simulink model "LoadFlow116BusNetwork_original"  (R2024a)
settings: Solver=FixedStepDiscrete  StartTime=0.0  StopTime=4.5  FixedStep=75e-6  RelTol=1e-3  EnableMultiTasking=on
undefined symbols (not defined in the file or in its folder): D1, D11, Delta
libraries: spsSeriesRLCBranchLib x164, spsLoadFlowBusLib x116, spsDistributedParametersLineLib x79, spsThreePhaseSeriesRLCLoadLib x60, spsThreePhaseTransformerTwoWindingsLib x52, spsThreePhaseParallelRLCLoadLib x44, spsThreePhaseVIMeasurementLib x44, spsSynchronousMachinepuStandardLib x28, spsExcitationSystemLib x28, spsHydraulicTurbineandGovernorLib x28, spsGenericPowerSystemStabilizerLib x28, spsMultiBandPowerSystemStabilizerLib x28
(part 8 of 15)

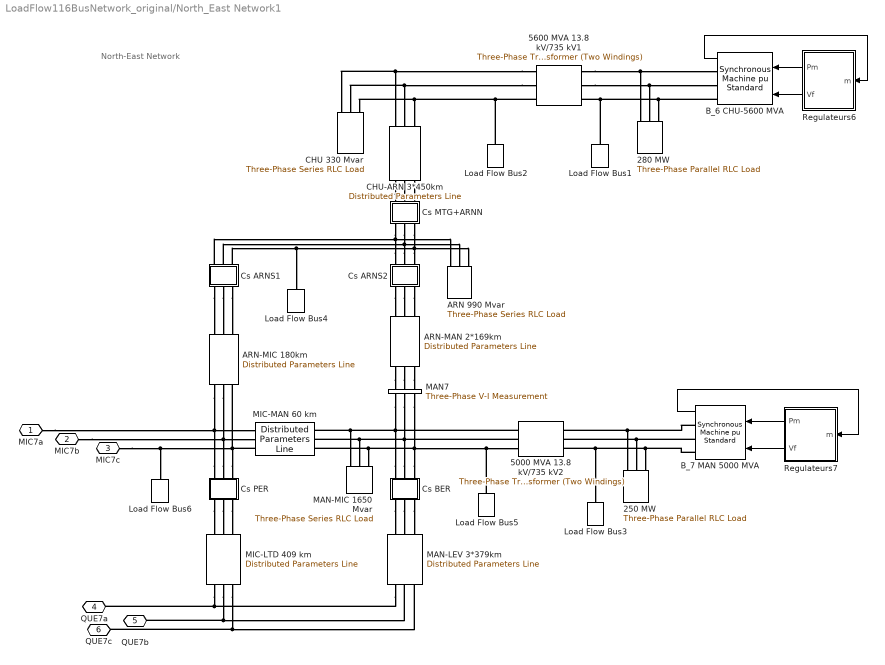
== system LoadFlow116BusNetwork_original/North_East Network1 ==
  note: North-East Network
  250 MW : spsThreePhaseParallelRLCLoadLib/Three-Phase Parallel RLC Load  LConnTagsString=A|B|C  Configuration=Y (grounded)  NominalVoltage=(13800)*1  Vabc=[1e3 1e3 1e3]  Vabcp=[1e3 1e3 1e3]  NominalFrequency=60  UnbalancedPower=off  ActivePower=250000000  InductivePower=0  CapacitivePower=0  Pabc=[10e3 9e3 11e3]  QLabc=[100 90 110]  QCabc=[100 90 110]  Pabcp=[10e3 9e3 11e3]  QLabcp=[100 90 110]  QCabcp=[100 90 110]  Measurements=None  LoadType=constant PQ
  280 MW : spsThreePhaseParallelRLCLoadLib/Three-Phase Parallel RLC Load  LConnTagsString=A|B|C  Configuration=Y (grounded)  NominalVoltage=(13800)*1  Vabc=[1e3 1e3 1e3]  Vabcp=[1e3 1e3 1e3]  NominalFrequency=60  UnbalancedPower=off  ActivePower=280000000  InductivePower=0  CapacitivePower=0  Pabc=[10e3 9e3 11e3]  QLabc=[100 90 110]  QCabc=[100 90 110]  Pabcp=[10e3 9e3 11e3]  QLabcp=[100 90 110]  QCabcp=[100 90 110]  Measurements=None  LoadType=constant PQ
  5000 MVA 13.8 kV/735 kV2 : spsThreePhaseTransformerTwoWindingsLib/Three-Phase Transformer (Two Windings)  Winding1Connection=Delta (D1)  Winding2Connection=Yg  CoreType=Three single-phase transformers  SetSaturation=off  Hysteresis=off  DataFile='basic_model'  SetInitialFlux=off  Measurements=None  UNITS=pu  NominalPower=[ 5000e6 60 ]  Winding1="[ 13.8e3 0.002  0.0]"  Winding2=[ 735e3 0.002 0.12]  Rm=500  Lm=500  L0=0.5  Saturation="[ 0,0  ;  0.005,1.2  ;  1.0,1.4 ]"  InitialFluxes=[ 0.8 , -0.8 , 0.7 ]  BreakLoop=off  DiscreteSolver=Trapezoidal iterative  DataType=off  TransfoNumber=0
  5600 MVA 13.8 kV/735 kV1 : spsThreePhaseTransformerTwoWindingsLib/Three-Phase Transformer (Two Windings)  Winding1Connection=Delta (D1)  Winding2Connection=Yg  CoreType=Three single-phase transformers  SetSaturation=off  Hysteresis=off  DataFile='basic_model'  SetInitialFlux=off  Measurements=None  UNITS=pu  NominalPower=[ 5600e6 60 ]  Winding1="[ 13.8e3 0.002  0.0]"  Winding2=[ 735e3 0.002 0.12]  Rm=500  Lm=500  L0=0.5  Saturation="[ 0,0  ;  0.005,1.2  ;  1.0,1.4 ]"  InitialFluxes=[ 0.8 , -0.8 , 0.7 ]  BreakLoop=off  DiscreteSolver=Trapezoidal iterative  DataType=off  TransfoNumber=0
  ARN 990 Mvar : spsThreePhaseSeriesRLCLoadLib/Three-Phase Series RLC Load  LConnTagsString=A|B|C  Configuration=Y (grounded)  NominalVoltage=735e3  Vabc=[1e3 1e3 1e3]  Vabcp=[1e3 1e3 1e3]  NominalFrequency=60  UnbalancedPower=off  ActivePower=3300000  InductivePower=990e6  CapacitivePower=0  Pabc=[10e3 9e3 11e3]  QLabc=[100 90 110]  QCabc=[100 90 110]  Pabcp=[10e3 9e3 11e3]  QLabcp=[100 90 110]  QCabcp=[100 90 110]  Measurements=None  LoadType=constant Z
  ARN-MAN 2*169km : spsDistributedParametersLineLib/Distributed Parameters Line  Phases=3  Length=169  Frequency=60  Resistance="[0.01273  0.3864]/2"  Inductance="[0.9337e-3  4.1264e-3]/2"  Capacitance=[12.74e-9 7.751e-9]*2  x1=[-0.000975 8.78499508384115e-10 336881.671287458 -573361.279314323;-0.0009 8.13651182104684e-10 352956.287913021 -563608.347624883;-0.000825 7.4815243551956e-10 368748.756682439 -553404.876045849;-0.00075 6.82055627324597e-10 384246.453337811 -542759.021076282;-0.000675 6.15413594296952e-10 399436.989257552 -531679.292849758;-0.0006 5.48279609058169e-10 414308.221359671 -520174.548331497;-0.000525 4.80707337488865e-10 428848.261808764 -508253.984238236;-0.00045 4.12750795829041e-10 443045.487518965 -495927.129686522;-0.000375 3.44464307498331e-10 456888.549445267 -483203.838575277;-0.0003 2.75902459670687e-10 470366.381655772 -470094.281708741;-0.000225 2.07120059638231e-10 483468.210177628 -456608.93866609;-0.00015 1.38172090999144e-10 496183.56160958 -442758.589424221;-7.5e-05 6.91136697046154e-11 508502.271494244 -428554.3057404]  x2=[-0.000975 3.53873333334227e-10 221203.742399991 -593985.664844307;-0.0009 3.00275393624317e-10 237907.645286788 -587494.731105826;-0.000825 2.46437418359111e-10 254421.368442051 -580534.163068269;-0.00075 1.92402444792288e-10 270731.71104816 -573109.524903227;-0.000675 1.38213667654954e-10 286825.63486679 -565226.751752846;-0.0006 8.39144046264366e-11 302690.274661488 -556892.144985374;-0.000525 2.95480617067942e-11 318312.948481937 -548112.367157935;-0.00045 -2.4841901481276e-11 333681.167801722 -538894.436690592;-0.000375 -7.9212006433396e-11 348782.647501459 -529245.722255919;-0.0003 -1.33518790519557e-10 363605.315689336 -519173.936888605;-0.000225 -1.87718841727484e-10 378137.3233512 -508687.131819771;-0.00015 -2.41768833365527e-10 392367.053822471 -497793.690040934;-7.5e-05 -2.95625558697366e-10 406283.132074335 -486502.319602777]  x3=[-0.000975 -3.60869348928103e-12 1173.57899596787 -608.93138738685;-0.0009 -3.82766651260744e-12 1190.32360835435 -575.511145378701;-0.000825 -4.04357975788894e-12 1206.11669426088 -541.630848566551;-0.00075 -4.25626062738083e-12 1220.94562893621 -507.317580341287;-0.000675 -4.46553910725016e-12 1234.79855835687 -472.598770204517;-0.0006 -4.6712479034822e-12 1247.66440870303 -437.50217184185;-0.000525 -4.87322257561268e-12 1259.53289521077 -402.05584093702;-0.00045 -5.07130166817902e-12 1270.39453039359 -366.288112744606;-0.000375 -5.26532683978534e-12 1280.2406316265 -330.227579439259;-0.0003 -5.45514298967813e-12 1289.06332808682 -293.903067259561;-0.000225 -5.64059838173146e-12 1296.855567046 -257.343613464762;-0.00015 -5.82154476574249e-12 1303.61111950744 -220.57844312285;-7.5e-05 -5.9978374959404e-12 1309.32458518586 -183.636945748468]  x4=[-0.000975 4.09065354206605e-12 1977.23728446549 -8416.68856749933;-0.0009 4.02816421017437e-12 2214.39295528562 -8357.4267304651;-0.000825 3.96245482544606e-12 2449.77847425865 -8291.48409437546;-0.00075 3.89357791495788e-12 2683.20567780222 -8218.91337276473;-0.000675 3.82158853785822e-12 2914.48796778139 -8139.77257755741;-0.0006 3.74654424135366e-12 3143.44046067226 -8054.12497269428;-0.000525 3.66850501470661e-12 3369.88013535513 -7962.03902356022;-0.00045 3.58753324128082e-12 3593.62597941869 -7863.58834225402;-0.000375 3.50369364867304e-12 3814.49913385863 -7758.85162874395;-0.0003 3.41705325697083e-12 4032.32303605475 -7647.91260795627;-0.000225 3.32768132517766e-12 4246.92356091246 -7530.85996284678;-0.00015 3.23564929584838e-12 4458.12916005569 -7407.78726350902;-7.5e-05 3.14103073797909e-12 4665.77099896003 -7278.79289237575]  x5=0.000955765248222805  V1=ones(3,3)  V2=ones(3,3)  I1=ones(3,3)  I2=ones(3,3)  nHarmo=1  Measurements=None  Decoupling=off  VsMag0=[ 1 1 1]  VrMag0=[ 1 1 1]  VsAngle0=[0 -120 120]  VrAngle0=[0 -120 120]  IsMag0=[ 1 1 1]  IrMag0=[ 1 1 1]  IsAngle0=[0 -120 120]  IrAngle0=[0 -120 120]
      settings: AttributesFormatString=\n  LibrarySourceBlock=sps_lib/Power Grid Elements/Distributed Parameters Line
  ARN-MIC 180km : spsDistributedParametersLineLib/Distributed Parameters Line  Phases=3  Length=180  Frequency=60  Resistance="[0.01273  0.3864]"  Inductance="[0.9337e-3  4.1264e-3]"  Capacitance=[12.74e-9 7.751e-9]  x1=[-0.00105 5.00976431216861e-10 327893.271560114 -568370.375306689;-0.000975 4.5408234490734e-10 343830.386178249 -558873.543002063;-0.0009 4.06825272118994e-10 359492.648046455 -548929.955738212;-0.000825 3.5924298943275e-10 374867.536992234 -538547.562266654;-0.00075 3.11373533397356e-10 389942.762564607 -527734.662113874;-0.000675 2.63255170123539e-10 404706.273858911 -516499.898946812;-0.0006 2.14926364694664e-10 419146.269150106 -504852.253663245;-0.000525 1.66425750418337e-10 433251.205326894 -492801.037212598;-0.00045 1.17792097943524e-10 447009.807119111 -480355.883152912;-0.000375 6.90642842678944e-11 460411.076110995 -467526.739949925;-0.0003 2.02812616601402e-11 473444.299533163 -454323.863024421;-0.000225 -2.85179734778713e-11 486099.058826224 -440757.806554203;-0.00015 -7.72944117842243e-11 498365.237969224 -426839.415037247;-7.5e-05 -1.26009062120441e-10 510233.031566236 -412579.814622772]  x2=[-0.00105 2.18032175619013e-09 183777.347501384 -621430.397175494;-0.000975 2.1855909220691e-09 201272.089254416 -615986.559734681;-0.0009 2.18911296000564e-09 218605.937178865 -610050.312062926;-0.000825 2.19088505453651e-09 235765.034861915 -603626.399505791;-0.00075 2.19090578907644e-09 252735.665583423 -596719.957240685;-0.000675 2.18917514705056e-09 269504.263280849 -589336.506171882;-0.0006 2.18569451190764e-09 286057.423393762 -581481.948517196;-0.000525 2.18046666601414e-09 302381.913579239 -573162.563089837;-0.00045 2.1734957884301e-09 318464.6842896 -564385.000279226;-0.000375 2.16478745156838e-09 334292.879204012 -555156.276734772;-0.0003 2.15434861674024e-09 349853.845505641 -545483.769756872;-0.000225 2.14218762859051e-09 365135.143996117 -535375.21139961;-0.00015 2.12831420842706e-09 380124.559039236 -524838.68228987;-7.5e-05 2.11273944644969e-09 394810.108325961 -513882.605167809]  x3=[-0.00105 -4.40575400200817e-12 35.6370942882288 24.8424671154528;-0.000975 -4.25272459462188e-12 34.9200556849036 25.839604901741;-0.0009 -4.09629562426352e-12 34.1751025233587 26.81608690323;-0.000825 -3.93659213785855e-12 33.4028303077532 27.7711325351485;-0.00075 -3.77374179993046e-12 32.6038563806801 28.7039783486309;-0.000675 -3.60787479054769e-12 31.778819429672 29.613878641007;-0.0006 -3.43912370125969e-12 30.9283789766441 30.500106051905;-0.000525 -3.26762342910525e-12 30.0532148506823 31.3619521446925;-0.00045 -3.09351106877791e-12 29.1540266445985 32.1987279727894;-0.000375 -2.91692580303449e-12 28.2315331556866 33.0097646304019;-0.0003 -2.73800879143459e-12 27.286471811127 33.7944137872352;-0.000225 -2.55690305749976e-12 26.3195980784985 34.5520482067589;-0.00015 -2.37375337438269e-12 25.3316848618695 35.2820622476101;-7.5e-05 -2.18870614913778e-12 24.3235218839497 35.9838723477343]  x4=[-0.00105 7.31127026918303e-12 1327.91429807013 -4613.1254825023;-0.000975 7.11574515856379e-12 1457.79983330337 -4573.74071492959;-0.0009 6.91453183013935e-12 1586.52002565494 -4530.69976900994;-0.000825 6.70779113076577e-12 1713.97197817258 -4484.03705101698;-0.00075 6.49568832579491e-12 1840.05380771551 -4433.7898624135;-0.000675 6.27839296696377e-12 1964.66472639833 -4379.99837003327;-0.0006 6.05607875685747e-12 2087.70512215924 -4322.70557397225;-0.000525 5.82892341005406e-12 2209.07663838846 -4261.95727321502;-0.00045 5.59710851106216e-12 2328.68225255295 -4197.80202902371;-0.000375 5.36081936916516e-12 2446.42635375479 -4130.29112611892;-0.0003 5.12024487028773e-12 2562.21481916101 -4059.47853168349;-0.000225 4.87557732600336e-12 2675.955089244 -3985.42085222194;-0.00015 4.62701231980343e-12 2787.55624177213 -3908.1772883101;-7.5e-05 4.3747485507507e-12 2896.92906449163 -3827.8095872711]  x5=0.00101797482059234  V1=ones(3,3)  V2=ones(3,3)  I1=ones(3,3)  I2=ones(3,3)  nHarmo=1  Measurements=None  Decoupling=off  VsMag0=[ 1 1 1]  VrMag0=[ 1 1 1]  VsAngle0=[0 -120 120]  VrAngle0=[0 -120 120]  IsMag0=[ 1 1 1]  IrMag0=[ 1 1 1]  IsAngle0=[0 -120 120]  IrAngle0=[0 -120 120]
      settings: AttributesFormatString=\n  LibrarySourceBlock=sps_lib/Power Grid Elements/Distributed Parameters Line
  "B_6 CHU-5600 MVA " : spsSynchronousMachinepuStandardLib/Synchronous Machine pu Standard  PresetModel=No  MechanicalLoad=Mechanical power Pm  ShowDetailedParameters=on  RotorType=Salient-pole  Units=per unit standard parameters  MeasurementBus=off  NominalParameters="[ 5600E6  13800   60 ]"  Reactances1=[ 31 32 33 34 35 36 37 ]  Reactances2=[ 1.305, 0.296, 0.252, 0.474, 0.243, 0.18 ]  dAxisTimeConstants=Short-circuit  qAxisTimeConstants=Open-circuit  TimeConstants1=[]  TimeConstants2=[]  TimeConstants3=[]  TimeConstants4=[]  TimeConstants5=[ 1.01, 0.053, 0.1 ]  TimeConstants6=[]  TimeConstants7=[]  TimeConstants8=[]  StatorResistance=2.8544e-3  Mechanical="[ 4.0 0  32]"  PolePairs=32  InitialConditions=[0 -61.7964 0.894782 0.894782 0.894782 8.48442 -111.516 128.484 1.31361]  SetSaturation=off  Saturation=[0.6404,0.7127,0.8441,0.9214,0.9956,1.082,1.19,1.316,1.457;0.7,0.7698,0.8872,0.9466,0.9969,1.046,1.1,1.151,1.201]  LoadFlowParameters=[1 5000000000 0 0 0]  TsPowergui=0  TsBlock=-1  IterativeModel=Trapezoidal non iterative  IterativeDiscreteModel=Trapezoidal non iterative  BusType=PV  Pref=5000000000  Qref=0  Qmin=-Inf  Qmax=Inf  PLF=0  QLF=0
  B_7 MAN 5000 MVA : spsSynchronousMachinepuStandardLib/Synchronous Machine pu Standard  PresetModel=No  MechanicalLoad=Mechanical power Pm  ShowDetailedParameters=on  RotorType=Salient-pole  Units=per unit standard parameters  MeasurementBus=off  NominalParameters="[ 5000E6  13800   60 ]"  Reactances1=[ 31 32 33 34 35 36 37 ]  Reactances2=[ 1.305, 0.296, 0.252, 0.474, 0.243, 0.18 ]  dAxisTimeConstants=Short-circuit  qAxisTimeConstants=Open-circuit  TimeConstants1=[]  TimeConstants2=[]  TimeConstants3=[]  TimeConstants4=[]  TimeConstants5=[ 1.01, 0.053, 0.1 ]  TimeConstants6=[]  TimeConstants7=[]  TimeConstants8=[]  StatorResistance=2.8544e-3  Mechanical="[ 3.7 0  32]"  PolePairs=32  InitialConditions=[0 -81.9543 0.907703 0.907703 0.907703 -8.76021 -128.76 111.24 1.25655]  SetSaturation=off  Saturation=[0.6404,0.7127,0.8441,0.9214,0.9956,1.082,1.19,1.316,1.457;0.7,0.7698,0.8872,0.9466,0.9969,1.046,1.1,1.151,1.201]  LoadFlowParameters=[1 4500000000 0 0 0]  TsPowergui=0  TsBlock=-1  IterativeModel=Trapezoidal non iterative  IterativeDiscreteModel=Trapezoidal non iterative  BusType=PV  Pref=4500000000  Qref=0  Qmin=-Inf  Qmax=Inf  PLF=0  QLF=0
  CHU 330 Mvar : spsThreePhaseSeriesRLCLoadLib/Three-Phase Series RLC Load  LConnTagsString=A|B|C  Configuration=Y (grounded)  NominalVoltage=735e3  Vabc=[1e3 1e3 1e3]  Vabcp=[1e3 1e3 1e3]  NominalFrequency=60  UnbalancedPower=off  ActivePower=1100000  InductivePower=330e6  CapacitivePower=0  Pabc=[10e3 9e3 11e3]  QLabc=[100 90 110]  QCabc=[100 90 110]  Pabcp=[10e3 9e3 11e3]  QLabcp=[100 90 110]  QCabcp=[100 90 110]  Measurements=None  LoadType=constant Z
  CHU-ARN 3*450km : spsDistributedParametersLineLib/Distributed Parameters Line  Phases=3  Length=450  Frequency=60  Resistance="[0.01273  0.3864]/3"  Inductance="[0.9337e-3  4.1264e-3]/3"  Capacitance=[12.74e-9 7.751e-9]*3  x1=[-0.00255 7.32999303821091e-10 0 0;-0.002475 6.56025529209857e-10 0 0;-0.0024 5.785273378281e-10 0 0;-0.002325 5.00566680544248e-10 0 0;-0.00225 4.22205877914896e-10 0 0;-0.002175 3.43507570366705e-10 0 0;-0.0021 2.64534668122606e-10 0 0;-0.002025 1.85350300912325e-10 0 0;-0.00195 1.0601776750745e-10 0 0;-0.001875 2.66004851213558e-11 0 0;-0.0018 -5.28380612855433e-11 0 0;-0.001725 -1.32234369754701e-10 0 0;-0.00165 -2.1152497209193e-10 0 0;-0.001575 -2.90646484602909e-10 351966.370721056 -543333.024589183;-0.0015 -3.69535658761137e-10 367186.081536598 -533165.672906027;-0.001425 -4.48129431767837e-10 382112.269416695 -522572.116741658;-0.00135 -5.26364976963391e-10 396733.002595135 -511560.824422788;-0.001275 -6.04179754050015e-10 411036.593481518 -500140.598208017;-0.0012 -6.81511559085512e-10 425011.608004143 -488320.567251446;-0.001125 -7.58298574208153e-10 438646.874750225 -476110.18030497;-0.00105 -8.34479417052929e-10 451931.493896154 -463519.198165088;-0.000975 -9.09993189819675e-10 464854.845920646 -450557.685870274;-0.0009 -9.84779527953843e-10 477406.600093827 -437236.00465514;-0.000825 -1.058778648401e-09 489576.722735458 -423564.803667819;-0.00075 -1.13193139739647e-09 501355.48523571 -409555.011457205;-0.000675 -1.20417929775201e-09 512733.471832061 -395217.827236834;-0.0006 -1.27546459560147e-09 523701.587136114 -380564.711932406;-0.000525 -1.34573030656848e-09 534251.063404314 -365607.379020094;-0.00045 -1.41492026131878e-09 544373.467546744 -350357.785162973;-0.000375 -1.48297915046119e-09 554060.70786841 -334828.120653048;-0.0003 -1.54985256876106e-09 563305.04053762 -319030.799666514;-0.000225 -1.61548705863101e-09 572099.075776279 -302978.450340062;-0.00015 -1.67983015286406e-09 580435.783767173 -286683.904676134;-7.5e-05 -1.74283041657518e-09 588308.500273488 -270160.188285219]  x2=[-0.00255 1.95007004339389e-09 0 0;-0.002475 1.90177200864104e-09 0 0;-0.0024 1.85195372644257e-09 0 0;-0.002325 1.80065502077103e-09 0 0;-0.00225 1.74791689902682e-09 0 0;-0.002175 1.69378151925756e-09 0 0;-0.0021 1.63829215645754e-09 0 0;-0.002025 1.58149316797435e-09 0 0;-0.00195 1.52342995805033e-09 0 0;-0.001875 1.46414894152712e-09 0 0;-0.0018 1.40369750674227e-09 0 0;-0.001725 1.34212397764783e-09 0 0;-0.00165 1.27947757518084e-09 0 0;-0.001575 1.21580837791692e-09 34511.8097316182 -640486.415414582;-0.0015 1.15116728203818e-09 52604.9373492512 -639254.768695381;-0.001425 1.08560596064763e-09 70656.0133848497 -637512.111495011;-0.00135 1.01917682246247e-09 88650.6080844217 -635259.836866974;-0.001275 9.51932969919355e-10 106574.336844291 -632499.745245147;-0.0012 8.83928156725153e-10 124412.871709928 -629234.043004542;-0.001125 8.15216744887019e-10 142151.952829502 -625465.340697562;-0.00105 7.45853661256256e-10 159777.399852982 -621196.65096717;-0.000975 6.75894353620629e-10 177275.123267695 -616431.386138622;-0.0009 6.05394746380248e-10 194631.135661268 -611173.355491711;-0.000825 5.34411195842461e-10 211831.56290295 -605426.762215686;-0.00075 4.63000445171483e-10 228862.655234379 -599196.200049286;-0.000675 3.91219579028779e-10 245710.79826093 -592486.649608576;-0.0006 3.1912597794046e-10 262362.523834852 -585303.474405518;-0.000525 2.46777272428167e-10 278804.520821502 -577652.416560464;-0.00045 1.74231296940113e-10 295023.645740059 -569539.592211991;-0.000375 1.01546043619113e-10 311006.933270225 -560971.48662775;-0.0003 2.87796159445515e-11 326741.6066165 -551954.949020251;-0.000225 -4.40098177146536e-11 342215.087721761 -542497.1870717;-0.00015 -1.1676407059895e-10 357415.007321963 -532605.761172288;-7.5e-05 -1.89424984071761e-10 372329.214833944 -522288.578376537]  x3=[-0.00255 4.87239052788349e-12 0 0;-0.002475 4.7899343714918e-12 0 0;-0.0024 4.703649214852e-12 0 0;-0.002325 4.61360403299809e-12 0 0;-0.00225 4.51987080667071e-12 0 0;-0.002175 4.42252446477682e-12 0 0;-0.0021 4.32164282449269e-12 0 0;-0.002025 4.217306529058e-12 0 0;-0.00195 4.10959898331094e-12 0 0;-0.001875 3.99860628701559e-12 0 0;-0.0018 3.88441716603514e-12 0 0;-0.001725 3.76712290140572e-12 0 0;-0.00165 3.64681725636784e-12 0 0;-0.001575 3.52359640141339e-12 -94.8473576352802 -855.378108345468;-0.0015 3.39755883740849e-12 -70.6281637624271 -857.719458194341;-0.001425 3.26880531685335e-12 -46.3525108161095 -859.375160231881;-0.00135 3.13743876334233e-12 -22.0398043818627 -860.343890915213;-0.001275 3.0035641892883e-12 2.29052033478661 -860.62487585585;-0.0012 2.86728861197744e-12 26.6190140445265 -860.21789043873;-0.001125 2.72872096802114e-12 50.9262289217237 -859.123260001768;-0.00105 2.58797202627384e-12 75.1927341507184 -857.341859575788;-0.000975 2.44515429928604e-12 99.3991314585203 -854.875113185033;-0.0009 2.3003819533635e-12 123.526070621492 -851.724992708825;-0.000825 2.15377071730447e-12 147.554264933621 -847.894016305276;-0.00075 2.00543778988782e-12 171.464506624018 -843.385246398306;-0.000675 1.85550174618617e-12 195.237682211315 -838.202287229592;-0.0006 1.70408244277874e-12 218.854787782689 -832.349281977391;-0.000525 1.55130092193989e-12 242.2969441853 -825.830909444549;-0.00045 1.39727931487974e-12 265.545412117997 -818.652380318334;-0.000375 1.24214074411436e-12 288.581607111227 -810.819433005094;-0.0003 1.08600922504354e-12 311.38711438318 -802.338329043062;-0.000225 9.29009566814706e-13 333.943703560277 -793.215848096982;-0.00015 7.71267272552487e-13 356.233343250259 -783.459282538543;-7.5e-05 6.12908439033376e-13 378.238215456199 -773.076431616971]  x4=[-0.00255 1.21136319031042e-11 0 0;-0.002475 1.18418780553791e-11 0 0;-0.0024 1.15606579915234e-11 0 0;-0.002325 1.12701965145533e-11 0 0;-0.00225 1.09707258149292e-11 0 0;-0.002175 1.06624852849464e-11 0 0;-0.0021 1.03457213273683e-11 0 0;-0.002025 1.00206871584559e-11 0 0;-0.00195 9.68764260555077e-12 0 0;-0.001875 9.34685389937263e-12 0 0;-0.0018 8.99859346119899e-12 0 0;-0.001725 8.64313968509556e-12 0 0;-0.00165 8.28077671537234e-12 0 0;-0.001575 7.91179421944299e-12 398.583364809259 -13326.9833161388;-0.0015 7.53648715626912e-12 775.187270557429 -13310.3877177131;-0.001425 7.15515554057465e-12 1151.17150346228 -13283.1519990016;-0.00135 6.76810420301859e-12 1526.23550748077 -13245.2979318211;-0.001275 6.37564254651811e-12 1900.07946218677 -13196.8557761338;-0.0012 5.97808429891655e-12 2272.40452244289 -13137.8642558577;-0.001125 5.57574726219419e-12 2642.91305729273 -13068.3705279116;-0.00105 5.16895305842222e-12 3011.30888788249 -12988.4301445182;-0.000975 4.75802687266299e-12 3377.29752422184 -12898.1070087969;-0.0009 4.343297193022e-12 3740.58640059472 -12797.4733236804;-0.000825 3.92509554805959e-12 4100.88510943186 -12686.6095341969;-0.00075 3.50375624177203e-12 4457.90563345816 -12565.6042631634;-0.000675 3.07961608635407e-12 4811.36257592932 -12434.5542403421;-0.0006 2.65301413295638e-12 5160.9733887736 -12293.5642251162;-0.000525 2.22429140065329e-12 5506.45859845643 -12142.7469227465;-0.00045 1.79379060383731e-12 5847.5420293873 -11982.222894277;-0.000375 1.36185587825854e-12 6183.95102469027 -11812.12046016;-0.0003 9.28832505927784e-13 6515.41666416172 -11632.5755976787;-0.000225 4.95066639103405e-13 6841.67397924106 -11443.731832249;-0.00015 6.09050235824992e-14 7162.46216482252 -11245.7401226875;-7.5e-05 -3.7330527848238e-13 7477.52478773877 -11038.7587405375]  x5=0.00254493705148084  V1=ones(3,3)  V2=ones(3,3)  I1=ones(3,3)  I2=ones(3,3)  nHarmo=1  Measurements=None  Decoupling=off  VsMag0=[ 1 1 1]  VrMag0=[ 1 1 1]  VsAngle0=[0 -120 120]  VrAngle0=[0 -120 120]  IsMag0=[ 1 1 1]  IrMag0=[ 1 1 1]  IsAngle0=[0 -120 120]  IrAngle0=[0 -120 120]
      settings: AttributesFormatString=\n  LibrarySourceBlock=sps_lib/Power Grid Elements/Distributed Parameters Line
  "Cs ARNS1 " : Subsystem  mask{Xc=25}
      mask prompts: Xc "Condensator Reactance at  60Hz  (ohm):"
      mask help: Series Compensation
      mask init:
      | Cs=1/Xc/(2*pi*60);
      mask Display: disp('Cs')
  Cs ARNS2 : Subsystem  mask{Xc=25/2}
      mask prompts: Xc "Condensator Reactance at  60Hz  (ohm):"
      mask help: Series Compensation
      mask init:
      | Cs=1/Xc/(2*pi*60);
      mask Display: disp('Cs')
  Cs BER : Subsystem  mask{Xc=22/3}
      mask prompts: Xc "Condensator Reactance at  60Hz  (ohm):"
      mask help: Series Compensation
      mask init:
      | Cs=1/Xc/(2*pi*60);
      mask Display: disp('Cs')
  "Cs MTG+ARNN " : Subsystem  mask{Xc=(30+25)/3}
      mask prompts: Xc "Condensator Reactance at  60Hz  (ohm):"
      mask help: Series Compensation
      mask init:
      | Cs=1/Xc/(2*pi*60);
      mask Display: disp('Cs')
  "Cs PER " : Subsystem  mask{Xc=22}
      mask prompts: Xc "Condensator Reactance at  60Hz  (ohm):"
      mask help: Series Compensation
      mask init:
      | Cs=1/Xc/(2*pi*60);
      mask Display: disp('Cs')
  Load Flow Bus1 : spsLoadFlowBusLib/Load Flow Bus  LConnTagsString=a  Phases=single  Connectors=on one side  ID=CHU_13.8  Vbase=13.8e3  Vref=1  Vangle=0  VLF=1  VLFb=1  VLFc=1  angleLF=4.726  angleLFb=0  angleLFc=0
      settings: AttributesFormatString=%<ID>\n%<Vbase>V\n%<VLF>pu\n%<angleLF>deg.
  Load Flow Bus2 : spsLoadFlowBusLib/Load Flow Bus  LConnTagsString=a  Phases=single  Connectors=on one side  ID=CHU7  Vbase=735e3  Vref=1  Vangle=0  VLF=1.009  VLFb=1  VLFc=1  angleLF=28.97  angleLFb=0  angleLFc=0
      settings: AttributesFormatString=%<ID>\n%<Vbase>V\n%<VLF>pu\n%<angleLF>deg.
  Load Flow Bus3 : spsLoadFlowBusLib/Load Flow Bus  LConnTagsString=a  Phases=single  Connectors=on one side  ID=MAN_13.8  Vbase=13.8e3  Vref=1  Vangle=0  VLF=1  VLFb=1  VLFc=1  angleLF=-16.23  angleLFb=0  angleLFc=0
      settings: AttributesFormatString=%<ID>\n%<Vbase>V\n%<VLF>pu\n%<angleLF>deg.
  Load Flow Bus4 : spsLoadFlowBusLib/Load Flow Bus  LConnTagsString=a  Phases=single  Connectors=on one side  ID=ARN7  Vbase=735e3  Vref=1  Vangle=0  VLF=1.054  VLFb=1  VLFc=1  angleLF=12.72  angleLFb=0  angleLFc=0
      settings: AttributesFormatString=%<ID>\n%<Vbase>V\n%<VLF>pu\n%<angleLF>deg.
  Load Flow Bus5 : spsLoadFlowBusLib/Load Flow Bus  LConnTagsString=a  Phases=single  Connectors=on one side  ID=MAN7  Vbase=735e3  Vref=1  Vangle=0  VLF=1.016  VLFb=1  VLFc=1  angleLF=7.996  angleLFb=0  angleLFc=0
      settings: AttributesFormatString=%<ID>\n%<Vbase>V\n%<VLF>pu\n%<angleLF>deg.
  Load Flow Bus6 : spsLoadFlowBusLib/Load Flow Bus  LConnTagsString=a  Phases=single  Connectors=on one side  ID=MIC7  Vbase=735e3  Vref=1  Vangle=0  VLF=1.041  VLFb=1  VLFc=1  angleLF=5.981  angleLFb=0  angleLFc=0
      settings: AttributesFormatString=%<ID>\n%<Vbase>V\n%<VLF>pu\n%<angleLF>deg.
  MAN-LEV 3*379km : spsDistributedParametersLineLib/Distributed Parameters Line  Phases=3  Length=379  Frequency=60  Resistance="[0.01273  0.3864]/3"  Inductance="[0.9337e-3  4.1264e-3]/3"  Capacitance=[12.74e-9 7.751e-9]*3  x1=[-0.002175 1.67803313912777e-09 2062.1369044793 -628964.364618995;-0.0021 1.66910605088395e-09 19842.5129723378 -628654.706299128;-0.002025 1.65884470480123e-09 37607.027238927 -627842.511025785;-0.00195 1.64725730364266e-09 55341.4790233482 -626528.428055441;-0.001875 1.63435311019944e-09 73031.6916761911 -624713.507845915;-0.0018 1.62014243988638e-09 90663.5239121303 -622399.201216655;-0.001725 1.60463665249587e-09 108222.881114253 -619587.358188969;-0.00165 1.58784814311713e-09 125695.726601078 -616280.226507151;-0.001575 1.56979033222767e-09 143068.092847268 -612480.449841668;-0.0015 1.55047765496523e-09 160326.09264905 -608191.065675846;-0.001425 1.5299255495885e-09 177455.930225441 -603415.502877758;-0.00135 1.50815044513609e-09 194443.912246376 -598157.578959236;-0.001275 1.48516974829331e-09 211276.458778952 -592421.497024212;-0.0012 1.4610018294776e-09 227940.11414302 -586211.84240882;-0.001125 1.43566600815348e-09 244421.557667442 -579533.579015948;-0.00105 1.40918253738887e-09 260707.61433844 -572392.045347172;-0.000975 1.38157258766509e-09 276785.265331495 -564792.950235238;-0.0009 1.3528582299535e-09 292641.658418402 -556742.368280507;-0.000825 1.32306241807232e-09 308264.118241136 -548246.734995017;-0.00075 1.29220897033765e-09 323640.156444348 -539312.841658028;-0.000675 1.26032255052356e-09 338757.481658358 -529947.829887181;-0.0006 1.22742864814616e-09 353604.009324694 -520159.185929596;-0.000525 1.19355355808773e-09 368167.871356299 -509954.734677481;-0.00045 1.15872435957694e-09 382437.425624699 -499342.633413034;-0.000375 1.12296889454218e-09 396401.265266543 -488331.365287635;-0.0003 1.08631574535512e-09 410048.227802076 -476929.732540546;-0.000225 1.04879421198242e-09 423367.404058252 -465146.849462533;-0.00015 1.01043428856374e-09 436348.146889362 -452992.135110045;-7.5e-05 9.71266639434954e-10 448980.0796882 -440475.305775763]  x2=[-0.002175 3.78299907288419e-09 -361248.126814298 -552999.635419983;-0.0021 3.99679302053708e-09 -345470.121722084 -562991.298925736;-0.002025 4.20739199300233e-09 -329415.953100435 -572532.915801182;-0.00195 4.41462764068364e-09 -313098.454406112 -581616.858623785;-0.001875 4.61833430257505e-09 -296530.669597903 -590235.86582864;-0.0018 4.81834913868786e-09 -279725.842709489 -598383.047513263;-0.001725 5.01451226022242e-09 -262697.407262361 -606051.890945271;-0.00165 5.20666685738078e-09 -245458.975527274 -613236.265768563;-0.001575 5.39465932471801e-09 -228024.327642798 -619930.42890383;-0.0015 5.57833938393212e-09 -210407.400599694 -626129.029139483;-0.001425 5.75756020399417e-09 -192622.277099891 -631827.111409339;-0.00135 5.93217851852278e-09 -174683.174298995 -637020.120753612;-0.001275 6.10205474030905e-09 -156604.432441306 -641703.90596009;-0.0012 6.26705307290048e-09 -138400.503396451 -645874.722882543;-0.001125 6.42704161915457e-09 -120085.93910678 -649529.237433737;-0.00105 6.58189248667534e-09 -101675.379954764 -652664.528250658;-0.000975 6.73148189004859e-09 -83183.5430596977 -655278.089029798;-0.0009 6.87569024979407e-09 -64625.21051306 -657367.830530658;-0.000825 7.01440228795544e-09 -46015.2175619372 -658932.082245856;-0.00075 7.14750712025178e-09 -27368.4407499517 -659969.593736507;-0.000675 7.27489834471672e-09 -8699.78602518191 -660479.535631798;-0.0006 7.39647412675457e-09 9975.8231754252 -660461.50029198;-0.000525 7.51213728054534e-09 28643.4578556211 -659915.502134229;-0.00045 7.62179534673359e-09 47288.1953938668 -658841.977621118;-0.000375 7.72536066633905e-09 65895.1314722483 -657241.784911716;-0.0003 7.82275045082982e-09 84449.3919907603 -655116.203175593;-0.000225 7.91388684830229e-09 102936.144957434 -652466.931570265;-0.00015 7.99869700571475e-09 121340.612344804 -649296.087882919;-7.5e-05 8.07711312712502e-09 139648.08190324 -645606.206837482]  x3=[-0.002175 -2.90270183723178e-11 -242.422201518429 1603.55585537922;-0.0021 -2.84802530716765e-11 -287.659078133579 1596.06084494432;-0.002025 -2.79107210924922e-11 -332.666004483001 1587.28996789051;-0.00195 -2.73188777099149e-11 -377.407002718399 1577.25023552273;-0.001875 -2.67051960344892e-11 -421.846307570345 1565.94967344941;-0.0018 -2.60701666339567e-11 -465.948394938484 1553.39731516697;-0.001725 -2.5414297141104e-11 -509.67801028896 1539.60319483856;-0.00165 -2.47381118479684e-11 -553.000196836344 1524.57833927291;-0.001575 -2.40421512867274e-11 -595.880323487565 1508.33475910968;-0.0015 -2.3326971797605e-11 -638.284112525465 1490.88543921831;-0.001425 -2.25931450841422e-11 -680.177667009886 1472.24432831814;-0.00135 -2.18412577561859e-11 -721.527497874367 1452.42632782801;-0.001275 -2.10719108609618e-11 -762.300550696787 1431.44727995429;-0.0012 -2.02857194026064e-11 -802.464232122571 1409.32395502684;-0.001125 -1.94833118505425e-11 -841.98643591931 1386.07403809312;-0.00105 -1.866532963709e-11 -880.835568642 1361.716114781;-0.000975 -1.78324266447147e-11 -918.980574888353 1336.26965644168;-0.0009 -1.69852686833248e-11 -956.390962124015 1309.75500458461;-0.000825 -1.61245329580329e-11 -993.036825057827 1282.1933546168;-0.00075 -1.52509075278079e-11 -1028.88886954766 1253.60673889952;-0.000675 -1.43650907554519e-11 -1063.91843601771 1224.01800913599;-0.0006 -1.34677907493393e-11 -1098.0975223685 1193.45081810407;-0.000525 -1.25597247973658e-11 -1131.39880636136 1161.92960074856;-0.00045 -1.16416187935594e-11 -1163.7956674594 1129.47955464833;-0.000375 -1.07142066578123e-11 -1195.26220810755 1096.12661987373;-0.0003 -9.7782297491957e-12 -1225.77327443466 1061.89745825051;-0.000225 -8.83443627332957e-12 -1255.30447636115 1026.81943204673;-0.00015 -7.88358068427795e-12 -1283.83220709603 990.920582099842;-7.5e-05 -6.92642308145014e-12 -1311.33366200786 954.229605401217]  x4=[-0.002175 3.85657296818227e-11 -6948.98880273993 -13531.9699054569;-0.0021 3.89006242920652e-11 -6563.65417562492 -13723.012784496;-0.002025 3.92044223384481e-11 -6173.07266378919 -13903.0856970842;-0.00195 3.94768809694614e-11 -5777.55649211721 -14072.0446956905;-0.001875 3.97177823858443e-11 -5377.42183018501 -14229.7547170766;-0.0018 3.99269340146903e-11 -4972.98853951908 -14376.0896902644;-0.001725 4.01041686633877e-11 -4564.57991790393 -14510.9326373154;-0.00165 4.02493446532698e-11 -4152.52244094282 -14634.1757668408;-0.001575 4.03623459328718e-11 -3737.14550107814 -14745.7205601686;-0.0015 4.04430821706996e-11 -3318.78114428015 -14845.4778500977;-0.001425 4.04914888274401e-11 -2897.76380461447 -14933.3678921768;-0.00135 4.05075272075524e-11 -2474.43003690066 -15009.3204284512;-0.001275 4.0491184490201e-11 -2049.1182476754 -15073.2747436253;-0.0012 4.04424737395041e-11 -1622.16842467551 -15125.1797135982;-0.001125 4.03614338940904e-11 -1193.92186505694 -15164.9938463311;-0.00105 4.02481297359723e-11 -764.720902567059 -15192.6853150154;-0.000975 4.01026518387604e-11 -334.908633888291 -15208.2319835148;-0.0009 3.99251164952598e-11 95.1713556281347 -15211.6214240602;-0.000825 3.97156656245075e-11 525.17526661904 -15202.850927185;-0.00075 3.94744666583252e-11 954.759360537262 -15181.9275038899;-0.000675 3.92017124074757e-11 1383.58023443098 -15148.8678800395;-0.0006 3.8897620907534e-11 1811.29509545478 -15103.6984829913;-0.000525 3.85624352445924e-11 2237.56203489302 -15046.45542047;-0.00045 3.81964233609413e-11 2662.04030147641 -14977.1844517042;-0.000375 3.77998778408804e-11 3084.39057377338 -14895.9409508463;-0.0003 3.73731156768309e-11 3504.27523143844 -14802.7898627078;-0.000225 3.69164780159373e-11 3921.35862510069 -14697.8056508433;-0.00015 3.64303298873588e-11 4335.30734467684 -14581.0722380255;-7.5e-05 3.5915059910471e-11 4745.79048589408 -14452.6829391585]  x5=0.00214340253891386  V1=ones(3,3)  V2=ones(3,3)  I1=ones(3,3)  I2=ones(3,3)  nHarmo=1  Measurements=None  Decoupling=off  VsMag0=[ 1 1 1]  VrMag0=[ 1 1 1]  VsAngle0=[0 -120 120]  VrAngle0=[0 -120 120]  IsMag0=[ 1 1 1]  IrMag0=[ 1 1 1]  IsAngle0=[0 -120 120]  IrAngle0=[0 -120 120]
      settings: AttributesFormatString=\n  LibrarySourceBlock=sps_lib/Power Grid Elements/Distributed Parameters Line
  MAN-MIC 1650 Mvar : spsThreePhaseSeriesRLCLoadLib/Three-Phase Series RLC Load  LConnTagsString=A|B|C  Configuration=Y (grounded)  NominalVoltage=735e3  Vabc=[1e3 1e3 1e3]  Vabcp=[1e3 1e3 1e3]  NominalFrequency=60  UnbalancedPower=off  ActivePower=5500000  InductivePower=1650e6  CapacitivePower=0  Pabc=[10e3 9e3 11e3]  QLabc=[100 90 110]  QCabc=[100 90 110]  Pabcp=[10e3 9e3 11e3]  QLabcp=[100 90 110]  QCabcp=[100 90 110]  Measurements=None  LoadType=constant Z
  MAN7 : spsThreePhaseVIMeasurementLib/Three-Phase V-I Measurement  VoltageMeasurement=no  SetLabelV=on  LabelV=Vabc_MAN7  Vpu=on  VpuLL=off  CurrentMeasurement=no  SetLabelI=on  LabelI=Iabc_MAN7  Ipu=on  Pbase=100e6  Vbase=735e3  OutputType=Magnitude  PhasorSimulation=off  PSBequivalent=0
  MIC-LTD 409 km : spsDistributedParametersLineLib/Distributed Parameters Line  Phases=3  Length=409  Frequency=60  Resistance="[0.01273  0.3864]"  Inductance="[0.9337e-3  4.1264e-3]"  Capacitance=[12.74e-9 7.751e-9]  x1=[-0.002325 1.53842757611934e-09 0 0;-0.00225 1.57333383342137e-09 0 0;-0.002175 1.60698239172977e-09 0 0;-0.0021 1.63934635290188e-09 0 0;-0.002025 1.67039984568232e-09 0 0;-0.00195 1.7001180463841e-09 0 0;-0.001875 1.72847719873227e-09 0 0;-0.0018 1.75545463285437e-09 0 0;-0.001725 1.78102878340232e-09 0 0;-0.00165 1.80517920679147e-09 0 0;-0.001575 1.82788659754288e-09 0 0;-0.0015 1.84913280371582e-09 0 0;-0.001425 1.86890084141815e-09 145223.563249275 -624254.194066337;-0.00135 1.88717490838299e-09 162813.550735164 -619899.168329356;-0.001275 1.90394039660082e-09 180273.387559726 -615048.604681987;-0.0012 1.91918390399686e-09 197589.116596549 -609706.380590595;-0.001125 1.93289324514455e-09 214746.895916779 -603876.766547379;-0.00105 1.94505746100633e-09 231733.00985415 -597564.42265661;-0.000975 1.95566682769416e-09 248533.879969079 -590774.394909411;-0.0009 1.96471286424263e-09 265136.075903055 -583512.111150073;-0.000825 1.97218833938855e-09 281526.326114673 -575783.376737116;-0.00075 1.97808727735145e-09 297691.528488693 -567594.369902577;-0.000675 1.98240496261058e-09 313618.760809671 -558951.636813223;-0.0006 1.98513794367442e-09 329295.291091786 -549862.086337647;-0.000525 1.98628403583971e-09 344708.587756589 -540332.984523424;-0.00045 1.98584232293792e-09 359846.329650558 -530371.948788746;-0.000375 1.98381315806758e-09 374696.415894438 -519986.941833169;-0.0003 1.98019816331204e-09 389246.975556499 -509186.265272357;-0.000225 1.97500022844279e-09 403486.377141979 -497978.553001898;-0.00015 1.96822350860945e-09 417403.23789112 -486372.764295497;-7.5e-05 1.95987342101815e-09 430986.432878374 -474378.17664307]  x2=[-0.002325 3.34651228385445e-09 0 0;-0.00225 3.56618105365427e-09 0 0;-0.002175 3.78299907288419e-09 0 0;-0.0021 3.99679302053708e-09 0 0;-0.002025 4.20739199300233e-09 0 0;-0.00195 4.41462764068364e-09 0 0;-0.001875 4.61833430257505e-09 0 0;-0.0018 4.81834913868786e-09 0 0;-0.001725 5.01451226022242e-09 0 0;-0.00165 5.20666685738078e-09 0 0;-0.001575 5.39465932471801e-09 0 0;-0.0015 5.57833938393212e-09 0 0;-0.001425 5.75756020399417e-09 -192622.277099891 -631827.111409339;-0.00135 5.93217851852278e-09 -174683.174298994 -637020.120753612;-0.001275 6.10205474030905e-09 -156604.432441306 -641703.90596009;-0.0012 6.26705307290048e-09 -138400.503396451 -645874.722882543;-0.001125 6.42704161915457e-09 -120085.93910678 -649529.237433737;-0.00105 6.58189248667534e-09 -101675.379954764 -652664.528250658;-0.000975 6.73148189004859e-09 -83183.5430596977 -655278.089029798;-0.0009 6.87569024979407e-09 -64625.21051306 -657367.830530658;-0.000825 7.01440228795544e-09 -46015.2175619372 -658932.082245856;-0.00075 7.14750712025178e-09 -27368.4407499517 -659969.593736507;-0.000675 7.27489834471672e-09 -8699.78602518191 -660479.535631798;-0.0006 7.39647412675457e-09 9975.8231754252 -660461.50029198;-0.000525 7.51213728054534e-09 28643.4578556211 -659915.502134229;-0.00045 7.62179534673359e-09 47288.1953938668 -658841.977621118;-0.000375 7.72536066633905e-09 65895.1314722483 -657241.784911716;-0.0003 7.82275045082982e-09 84449.3919907603 -655116.203175593;-0.000225 7.91388684830229e-09 102936.144957434 -652466.931570265;-0.00015 7.99869700571475e-09 121340.612344804 -649296.087882919;-7.5e-05 8.07711312712502e-09 139648.08190324 -645606.206837482]  x3=[-0.002325 -8.48513157402571e-12 0 0;-0.00225 -8.28929231472093e-12 0 0;-0.002175 -8.08682672197019e-12 0 0;-0.0021 -7.8778966436705e-12 0 0;-0.002025 -7.66266909532972e-12 0 0;-0.00195 -7.44131612655691e-12 0 0;-0.001875 -7.21401468352848e-12 0 0;-0.0018 -6.98094646754016e-12 0 0;-0.001725 -6.74229778975775e-12 0 0;-0.00165 -6.49825942228283e-12 0 0;-0.001575 -6.24902644565244e-12 0 0;-0.0015 -5.99479809289471e-12 0 0;-0.001425 -5.73577759026499e-12 -230.757724949418 15.8712450237451;-0.00135 -5.47217199478997e-12 -231.114329922699 9.34106728383541;-0.001275 -5.20419202874934e-12 -231.286185636807 2.80342243766211;-0.0012 -4.93205191122775e-12 -231.273154712914 -3.73646342151407;-0.001125 -4.65596918687124e-12 -231.075247567742 -10.2733624090009;-0.00105 -4.37616455198547e-12 -230.692622405235 -16.8020490277657;-0.000975 -4.0928616781144e-12 -230.125585090091 -23.3173043456176;-0.0009 -3.80628703324073e-12 -229.374588903267 -29.8139201671424;-0.000825 -3.51666970075083e-12 -228.440234179622 -36.2867031970539;-0.00075 -3.224241196309e-12 -227.323267828027 -42.7304791916348;-0.000675 -2.92923528278739e-12 -226.024582734292 -49.1400970949481;-0.0006 -2.63188778339952e-12 -224.545217047412 -55.5104331565125;-0.000525 -2.33243639318683e-12 -222.886353349681 -61.8363950271497;-0.00045 -2.03112048900891e-12 -221.049317711358 -68.1129258297307;-0.000375 -1.72818093818925e-12 -219.035578630624 -74.3350082015661;-0.0003 -1.42385990596966e-12 -216.84674585969 -80.497668305209;-0.000225 -1.11840066192703e-12 -214.484569117983 -86.5959798044643;-0.00015 -8.12047385507357e-13 -211.950936693446 -92.6250678024269;-7.5e-05 -5.05044970832451e-13 -209.247873933074 -98.5801127383993]  x4=[-0.002325 8.64345601180624e-12 0 0;-0.00225 8.81180356965326e-12 0 0;-0.002175 8.9731071065518e-12 0 0;-0.0021 9.12723767892252e-12 0 0;-0.002025 9.27407207714412e-12 0 0;-0.00195 9.41349292404531e-12 0 0;-0.001875 9.54538876873429e-12 0 0;-0.0018 9.66965417569089e-12 0 0;-0.001725 9.78618980905012e-12 0 0;-0.00165 9.89490251200971e-12 0 0;-0.001575 9.99570538129829e-12 0 0;-0.0015 1.00885178366445e-11 0 0;-0.001425 1.01732656851916e-11 -1193.29181621035 -4540.40590051556;-0.00135 1.02498811808061e-11 -1064.45477492595 -4572.32612353436;-0.001275 1.03183030782331e-11 -934.766824781183 -4600.59129900895;-0.0012 1.03784766820547e-11 -804.331636339096 -4625.17883219051;-0.001125 1.04303538904127e-11 -673.253477493606 -4646.06906818123;-0.00105 1.04738932334605e-11 -541.637130119331 -4663.24530764609;-0.000975 1.05090599065134e-11 -409.587806310565 -4676.69382016206;-0.0009 1.0535825797871e-11 -277.211064276338 -4686.40385519401;-0.000825 1.05541695112893e-11 -144.6127239588 -4692.3676506885;-0.00075 1.05640763830846e-11 -11.8987824423782 -4694.58043927866;-0.000675 1.0565538493855e-11 120.824670778671 -4693.04045209515;-0.0006 1.05585546748115e-11 253.451538606579 -4687.74892018016;-0.000525 1.05431305087123e-11 385.875801152463 -4678.71007350335;-0.00045 1.05192783253998e-11 517.991600487004 -4665.93113758044;-0.000375 1.04870171919443e-11 649.693325261652 -4649.42232769729;-0.0003 1.04463728974022e-11 780.875695132728 -4629.19684074393;-0.000225 1.03973779322009e-11 911.433844920914 -4605.27084466516;-0.00015 1.03400714621658e-11 1041.26340843887 -4577.66346553617;-7.5e-05 1.02744992972122e-11 1170.26060191999 -4546.39677227344]  x5=0.00231306500901259  V1=ones(3,3)  V2=ones(3,3)  I1=ones(3,3)  I2=ones(3,3)  nHarmo=1  Measurements=None  Decoupling=off  VsMag0=[ 1 1 1]  VrMag0=[ 1 1 1]  VsAngle0=[0 -120 120]  VrAngle0=[0 -120 120]  IsMag0=[ 1 1 1]  IrMag0=[ 1 1 1]  IsAngle0=[0 -120 120]  IrAngle0=[0 -120 120]
      settings: AttributesFormatString=\n  LibrarySourceBlock=sps_lib/Power Grid Elements/Distributed Parameters Line
  MIC-MAN 60 km : spsDistributedParametersLineLib/Distributed Parameters Line  Phases=3  Length=60  Frequency=60  Resistance="[0.01273  0.3864]"  Inductance="[0.9337e-3  4.1264e-3]"  Capacitance=[12.74e-9 7.751e-9]  x1=[-0.000375 2.16478745156838e-09 334292.879204012 -555156.276734772;-0.0003 2.15434861674024e-09 349853.845505641 -545483.769756872;-0.000225 2.14218762859051e-09 365135.143996117 -535375.21139961;-0.00015 2.12831420842706e-09 380124.559039236 -524838.68228987;-7.5e-05 2.11273944644969e-09 394810.108325961 -513882.605167809]  x2=[-0.000375 -7.9212006433396e-11 348782.647501459 -529245.722255919;-0.0003 -1.33518790519557e-10 363605.315689336 -519173.936888605;-0.000225 -1.87718841727484e-10 378137.3233512 -508687.131819771;-0.00015 -2.41768833365527e-10 392367.053822471 -497793.690040934;-7.5e-05 -2.95625558697366e-10 406283.132074335 -486502.319602777]  x3=[-0.000375 1.31847001726371e-11 2401.79476190193 -2735.13228390529;-0.0003 1.24911906002742e-11 2478.158487281 -2666.13912589987;-0.000225 1.1787695761267e-11 2552.54121068242 -2595.01469707051;-0.00015 1.1074778018626e-11 2624.88347169522 -2521.81585319736;-7.5e-05 1.03530072678868e-11 2695.1274410228 -2446.60110831624]  x4=[-0.000375 -1.14931518764036e-11 -40.0475234768889 -1360.36447471847;-0.0003 -1.08893687156409e-11 -1.57321375627302 -1360.95300908529;-0.000225 -1.02768807601399e-11 36.9023535673487 -1360.45361843992;-0.00015 -9.6561776234007e-12 75.3484217141535 -1358.86670198762;-7.5e-05 -9.02775548601387e-12 113.73425748551 -1356.1935282851]  x5=0.000339324940197445  V1=ones(3,3)  V2=ones(3,3)  I1=ones(3,3)  I2=ones(3,3)  nHarmo=1  Measurements=None  Decoupling=off  VsMag0=[ 1 1 1]  VrMag0=[ 1 1 1]  VsAngle0=[0 -120 120]  VrAngle0=[0 -120 120]  IsMag0=[ 1 1 1]  IrMag0=[ 1 1 1]  IsAngle0=[0 -120 120]  IrAngle0=[0 -120 120]
      settings: AttributesFormatString=\n  LibrarySourceBlock=sps_lib/Power Grid Elements/Distributed Parameters Line
  Regulateurs6 : Subsystem
  Regulateurs7 : Subsystem
  "MIC7a " : PMIOPort  Side=Left
  MIC7b : PMIOPort  Port=2  Side=Left
  MIC7c : PMIOPort  Port=3  Side=Left
  QUE7a : PMIOPort  Port=4  Side=Left
  QUE7b : PMIOPort  Port=5  Side=Left
  QUE7c : PMIOPort  Port=6  Side=Left
  wires:
  Regulateurs6/1(Pm) -> "B_6 CHU-5600 MVA "/1
  Regulateurs6/2(Vf) -> "B_6 CHU-5600 MVA "/2
  "B_6 CHU-5600 MVA "/1 -> Regulateurs6/1(m)
  Regulateurs7/1(Pm) -> B_7 MAN 5000 MVA/1
  Regulateurs7/2(Vf) -> B_7 MAN 5000 MVA/2
  B_7 MAN 5000 MVA/1 -> Regulateurs7/1(m)
  connections:
  "Cs PER "/RConn3 -- MIC-LTD 409 km/LConn3
  "Cs PER "/RConn2 -- MIC-LTD 409 km/LConn2
  "Cs PER "/RConn1 -- MIC-LTD 409 km/LConn1
  Cs BER/RConn3 -- MAN-LEV 3*379km/LConn3
  Cs BER/RConn2 -- MAN-LEV 3*379km/LConn2
  Cs BER/RConn1 -- MAN-LEV 3*379km/LConn1
  Cs ARNS2/RConn3 -- ARN-MAN 2*169km/LConn3
  Cs ARNS2/RConn2 -- ARN-MAN 2*169km/LConn2
  Cs ARNS2/RConn1 -- ARN-MAN 2*169km/LConn1
  CHU-ARN 3*450km/RConn3 -- "Cs MTG+ARNN "/LConn3
  CHU-ARN 3*450km/RConn2 -- "Cs MTG+ARNN "/LConn2
  CHU-ARN 3*450km/RConn1 -- "Cs MTG+ARNN "/LConn1
  Load Flow Bus2/LConn1 -- 5600 MVA 13.8 kV/735 kV1/RConn3 -- CHU-ARN 3*450km/LConn3 -- CHU 330 Mvar/LConn3
  5600 MVA 13.8 kV/735 kV1/RConn2 -- CHU-ARN 3*450km/LConn2 -- CHU 330 Mvar/LConn2
  5600 MVA 13.8 kV/735 kV1/RConn1 -- CHU-ARN 3*450km/LConn1 -- CHU 330 Mvar/LConn1
  "B_6 CHU-5600 MVA "/RConn3 -- Load Flow Bus1/LConn1 -- 5600 MVA 13.8 kV/735 kV1/LConn3 -- 280 MW/LConn3
  5600 MVA 13.8 kV/735 kV1/LConn2 -- "B_6 CHU-5600 MVA "/RConn2 -- 280 MW/LConn2
  5600 MVA 13.8 kV/735 kV1/LConn1 -- "B_6 CHU-5600 MVA "/RConn1 -- 280 MW/LConn1
  "Cs ARNS1 "/RConn1 -- ARN-MIC 180km/LConn1
  "Cs ARNS1 "/RConn2 -- ARN-MIC 180km/LConn2
  "Cs ARNS1 "/RConn3 -- ARN-MIC 180km/LConn3
  "Cs PER "/LConn3 -- Load Flow Bus6/LConn1 -- MIC7c/RConn1 -- MIC-MAN 60 km/LConn3 -- ARN-MIC 180km/RConn3
  "Cs PER "/LConn2 -- MIC7b/RConn1 -- ARN-MIC 180km/RConn2 -- MIC-MAN 60 km/LConn2
  "Cs PER "/LConn1 -- "MIC7a "/RConn1 -- ARN-MIC 180km/RConn1 -- MIC-MAN 60 km/LConn1
  ARN-MAN 2*169km/RConn1 -- MAN7/LConn1
  ARN-MAN 2*169km/RConn2 -- MAN7/LConn2
  ARN-MAN 2*169km/RConn3 -- MAN7/LConn3
  Cs BER/LConn1 -- 5000 MVA 13.8 kV/735 kV2/RConn1 -- MIC-MAN 60 km/RConn1 -- MAN-MIC 1650 Mvar/LConn1 -- MAN7/RConn1
  Cs BER/LConn2 -- 5000 MVA 13.8 kV/735 kV2/RConn2 -- MIC-MAN 60 km/RConn2 -- MAN-MIC 1650 Mvar/LConn2 -- MAN7/RConn2
  Cs BER/LConn3 -- Load Flow Bus5/LConn1 -- 5000 MVA 13.8 kV/735 kV2/RConn3 -- MIC-MAN 60 km/RConn3 -- MAN-MIC 1650 Mvar/LConn3 -- MAN7/RConn3
  B_7 MAN 5000 MVA/RConn1 -- 5000 MVA 13.8 kV/735 kV2/LConn1 -- 250 MW/LConn1
  B_7 MAN 5000 MVA/RConn2 -- 5000 MVA 13.8 kV/735 kV2/LConn2 -- 250 MW/LConn2
  B_7 MAN 5000 MVA/RConn3 -- 5000 MVA 13.8 kV/735 kV2/LConn3 -- Load Flow Bus3/LConn1 -- 250 MW/LConn3
  MIC-LTD 409 km/RConn2 -- MAN-LEV 3*379km/RConn2 -- QUE7b/RConn1
  Cs ARNS2/LConn1 -- ARN 990 Mvar/LConn1 -- "Cs MTG+ARNN "/RConn1 -- "Cs ARNS1 "/LConn1
  Cs ARNS2/LConn2 -- ARN 990 Mvar/LConn2 -- "Cs MTG+ARNN "/RConn2 -- "Cs ARNS1 "/LConn2
  Cs ARNS2/LConn3 -- Load Flow Bus4/LConn1 -- "Cs ARNS1 "/LConn3 -- ARN 990 Mvar/LConn3 -- "Cs MTG+ARNN "/RConn3
  MIC-LTD 409 km/RConn1 -- QUE7a/RConn1 -- MAN-LEV 3*379km/RConn1
  MIC-LTD 409 km/RConn3 -- QUE7c/RConn1 -- MAN-LEV 3*379km/RConn3
